simulink model "io302"  (Simulink 6.0)
settings: Solver=FixedStepDiscrete  StartTime=0.0  StopTime=inf  RelTol=1e-3
libraries: xpcdiamondlib x2
settings Model: Creator=ekbas  LastModifiedBy=ekbas  ExtModeArmWhenConnect=off  BufferReuse=off
settings DataIOCC: SaveFormat=Structure  SignalLoggingName=sigsOut
settings OptimizationCC: InlineInvariantSignals=off  OptimizeBlockIOStorage=off  BufferReuse=off  LocalBlockOutputs=off
settings DebuggingCC: CheckExecutionContextPreStartOutputMsg=on  CheckExecutionContextRuntimeOutputMsg=on  SolverPrmCheckMsg=none
settings RTWCC: SystemTargetFile=xpctarget.tlc  TemplateMakefile=xpc_default_tmf  ProcessScript=xpctarget_make_rtw_hook
settings xpcTargetCC: TargetFcnLib=ansi_tfl_tmw.mat  GenFloatMathFcnCalls=ANSI_C  ModelReferenceCompliant=off  LifeSpan=inf
settings SFSimCC: SFSimApplyToAllLibs=on  SFSimBuildMode=Incremental

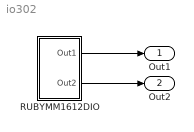
== system io302 ==
  RUBYMM1612DIO : Subsystem  PropExecContextAcrossSSBoundary=on
  Out1 : Outport
  Out2 : Outport  Port=2
  wires:
  RUBYMM1612DIO/1(Out1) -> Out1/1
  RUBYMM1612DIO/2(Out2) -> Out2/1

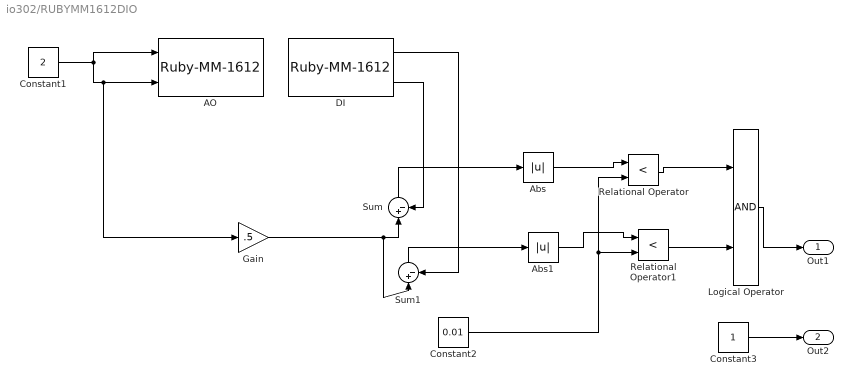
== system io302/RUBYMM1612DIO ==
  AO : xpcdiamondlib/D//A/Ruby-MM-1612   channel=[2,4]  range1=-10V to 10V  range2=-10V to 10V  reset=[1]  initValue=[0]  sampleTime=.001  base=0x300
  Abs : Abs  SaturateOnIntegerOverflow=on
  Abs1 : Abs  SaturateOnIntegerOverflow=on
  Constant1 : Constant  Value=2
  Constant2 : Constant  Value=0.01
  Constant3 : Constant
  DI : xpcdiamondlib/Digital Input/Ruby-MM-1612   channel=[3,5]  port=C  chip=1  sampletime=.001  baseaddress=0x300
  Gain : Gain  Gain=.5  SaturateOnIntegerOverflow=on
  Logical Operator : Logic  AllPortsSameDT=off
  Relational Operator : RelationalOperator  Operator=<
  Relational Operator1 : RelationalOperator  Operator=<
  Sum : Sum  Orientation=up  Inputs=|+-  SaturateOnIntegerOverflow=on
  Sum1 : Sum  Orientation=up  Inputs=|+-  SaturateOnIntegerOverflow=on
  Out1 : Outport
  Out2 : Outport  Port=2
  wires:
  Constant1/1 -> AO/1, AO/2, Gain/1
  Abs1/1 -> Relational Operator1/1
  Constant2/1 -> Relational Operator/2, Relational Operator1/2
  DI/2 -> Sum/2
  DI/1 -> Sum1/2
  Relational Operator1/1 -> Logical Operator/2
  Relational Operator/1 -> Logical Operator/1
  Abs/1 -> Relational Operator/1
  Sum1/1 -> Abs1/1
  Sum/1 -> Abs/1
  Gain/1 -> Sum/1, Sum1/1
  Logical Operator/1 -> Out1/1
  Constant3/1 -> Out2/1
